simulink model "ramp_ball_animation"  (R2015a)
settings: Solver=ode45  StartTime=0.0  StopTime=inf  RelTol=1e-3
undefined symbols (not defined in the file or in its folder): drawRamp
libraries: simulink x2
settings Model: Creator=ecestudent  LastModifiedBy=ecestudent

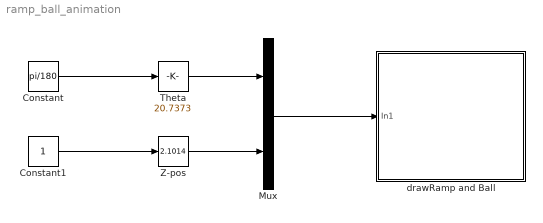
== system ramp_ball_animation ==
  Constant : Constant  Value=pi/180
  Constant1 : Constant
  Mux : Mux  Inputs=2
  Theta : simulink/Math Operations/Slider Gain  low=0  gain=20.7373  high=90
  Z-pos : simulink/Math Operations/Slider Gain  low=0  gain=2.1014  high=3
  drawRamp and Ball : Subsystem
      mask Display: image(imread('tv.jpg'))
  wires:
  Constant/1 -> Theta/1
  Constant1/1 -> Z-pos/1
  Theta/1 -> Mux/1
  Z-pos/1 -> Mux/2
  Mux/1 -> drawRamp and Ball/1(In1)

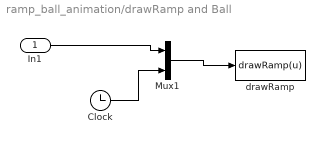
== system ramp_ball_animation/drawRamp and Ball ==
  In1 : Inport
  Clock : Clock
  Mux1 : Mux  Inputs=2
  drawRamp : MATLABFcn  MATLABFcn=drawRamp(u)  OutputDimensions=0
  wires:
  In1/1 -> Mux1/1
  Clock/1 -> Mux1/2
  Mux1/1 -> drawRamp/1
